simulink model "problem7"  (R2020b)
settings: Solver=FixedStepAuto  StartTime=0.0  StopTime=10.0  RelTol=1e-3
settings Model: Creator=Administrator  LastModifiedBy=Administrator

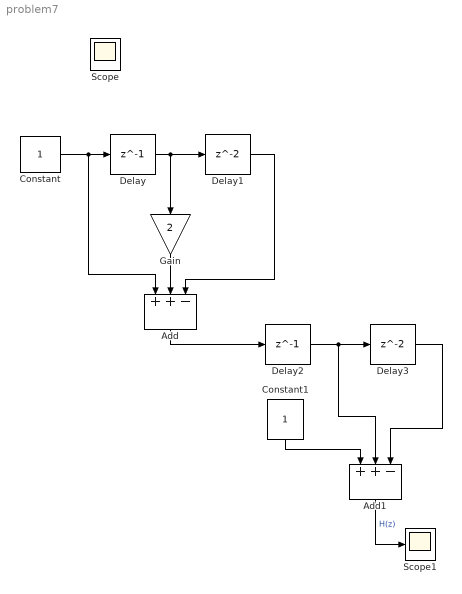
== system problem7 ==
  Add : Sum  Inputs=++-
  Add1 : Sum  Inputs=++-
  Constant : Constant
  Constant1 : Constant
  Delay : Delay  DelayLength=1
  Delay1 : Delay
  Delay2 : Delay  DelayLength=1
  Delay3 : Delay
  Gain : Gain  Gain=2
  Scope1 : Scope
  Scope : Scope
  wires:
  Delay1/1 -> Add/3
  Delay3/1 -> Add1/3
  Delay2/1 -> Delay3/1, Add1/2
  Add/1 -> Delay2/1
  Gain/1 -> Add/2
  Delay/1 -> Delay1/1, Gain/1
  Constant/1 -> Add/1, Delay/1
  Add1/1 -> Scope1/1  "H(z)"
  Constant1/1 -> Add1/1
